simulink model "SimplifiedDCMotor_noL_openLoop"  (R2020a)
settings: Solver=ode23  StartTime=0.0  StopTime=15  MaxStep=0.2  RelTol=1e-3
libraries: fmu_me_lib x1
settings Model: Creator=Bob  LastModifiedBy=meagh
settings DebuggingCC: ArithmeticOperatorsInVariantConditions=warning
settings SFSimCC: CustomCodeUndefinedFunction=UseInterfaceOnly
settings RTWCC: Description=FMU Model Exchange 1.0  SystemTargetFile=fmu_me1.tlc  MakeCommand=make_rtw FMIT_INTERMEDIATE_LIB_DIR=DEFAULT  TemplateMakefile=fmu_me1_default_tmf
settings STFCustomTargetCC: TargetLangStandard=C99 (ISO)  ModelReferenceCompliant=off  MATLABClassNameForMDSCustomization=Simulink.SoftwareTarget.TargetSpecificTriggerConfigurationBase  GRTInterface=on  SystemTargetFile=fmu_me1.tlc

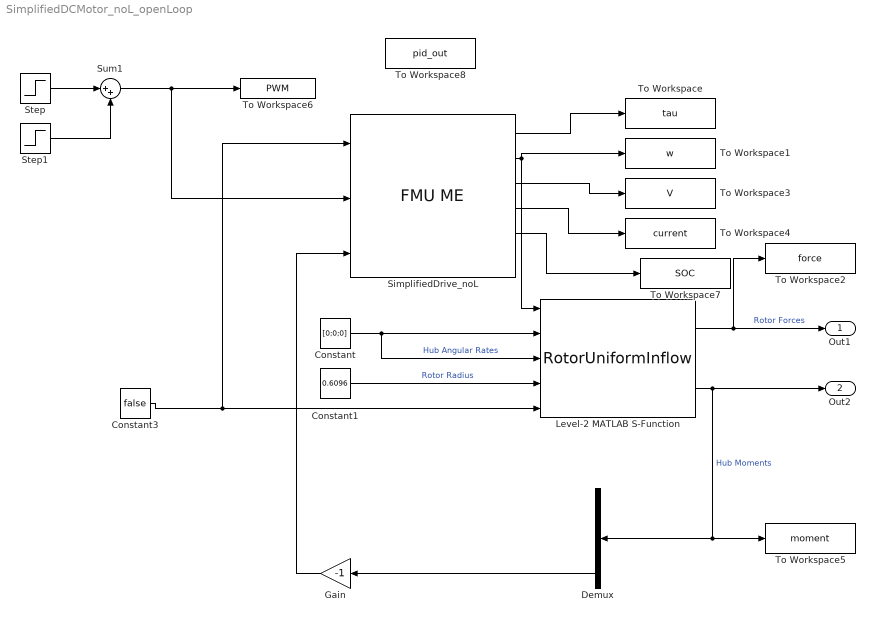
== system SimplifiedDCMotor_noL_openLoop ==
  Constant : Constant  Value=[0;0;0]
  Constant1 : Constant  Value=0.6096
  Constant3 : Constant  Value=false  OutDataTypeStr=boolean
  Demux : Demux  Outputs=3
  Gain : Gain  Gain=-1
  Level-2 MATLAB S-Function : M-S-Function  FunctionName=RotorUniformInflow
  SimplifiedDrive_noL : fmu_me_lib/FMU ME  Description=Simulates an FMU for Model Exchange 1.0 or Model Exchange 2.0.  dummy=0
  Step : Step  Time=5  After=0.5  SampleTime=0
  Step1 : Step  Time=10  After=0.2  SampleTime=0
  Sum1 : Sum  Inputs=|++
  To Workspace : ToWorkspace  VariableName=tau  SaveFormat=Timeseries  SampleTime=-1
  To Workspace1 : ToWorkspace  VariableName=w  SaveFormat=Timeseries  SampleTime=-1
  To Workspace2 : ToWorkspace  VariableName=force  SaveFormat=Timeseries  SampleTime=-1
  To Workspace3 : ToWorkspace  VariableName=V  SaveFormat=Timeseries  SampleTime=-1
  To Workspace4 : ToWorkspace  VariableName=current  SaveFormat=Timeseries  SampleTime=-1
  To Workspace5 : ToWorkspace  VariableName=moment  SaveFormat=Timeseries  SampleTime=-1
  To Workspace6 : ToWorkspace  VariableName=PWM  SaveFormat=Timeseries  SampleTime=-1
  To Workspace7 : ToWorkspace  VariableName=SOC  SaveFormat=Timeseries  SampleTime=-1
  To Workspace8 : ToWorkspace  VariableName=pid_out  SaveFormat=Timeseries  SampleTime=-1
  Out1 : Outport  OutDataTypeStr=double  VectorParamsAs1DForOutWhenUnconnected=off
  Out2 : Outport  Port=2  OutDataTypeStr=double  VectorParamsAs1DForOutWhenUnconnected=off
  wires:
  Level-2 MATLAB S-Function/1 -> To Workspace2/1, Out1/1  "Rotor Forces"
  Level-2 MATLAB S-Function/2 -> To Workspace5/1, Demux/1, Out2/1  "Hub Moments"
  Constant1/1 -> Level-2 MATLAB S-Function/4  "Rotor Radius"
  Constant/1 -> Level-2 MATLAB S-Function/3, Level-2 MATLAB S-Function/2  "Hub Angular Rates"
  Demux/3 -> Gain/1
  Constant3/1 -> SimplifiedDrive_noL/1, Level-2 MATLAB S-Function/5
  SimplifiedDrive_noL/2 -> Level-2 MATLAB S-Function/1, To Workspace1/1
  Gain/1 -> SimplifiedDrive_noL/3
  SimplifiedDrive_noL/1 -> To Workspace/1
  Step/1 -> Sum1/1
  Step1/1 -> Sum1/2
  SimplifiedDrive_noL/3 -> To Workspace3/1
  SimplifiedDrive_noL/4 -> To Workspace4/1
  SimplifiedDrive_noL/5 -> To Workspace7/1
  Sum1/1 -> To Workspace6/1, SimplifiedDrive_noL/2
